simulink model "successPIDCloseLoop21picont"  (R2023b)
settings: Solver=FixedStepAuto  StartTime=0.0  StopTime=inf  RelTol=1e-3  EnableMultiTasking=on
libraries: arduinolib x5, simulink x1, arduinosensorlib x1, slpidlib x1
(part 3 of 3)

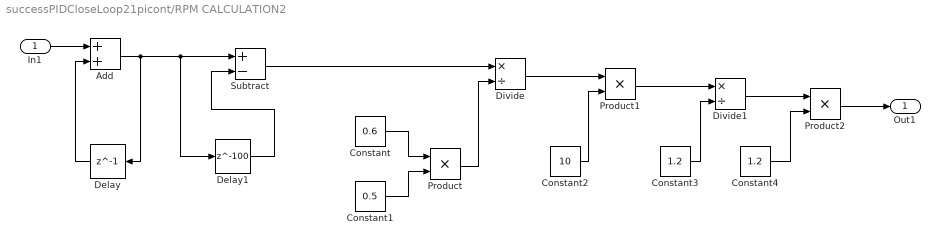
== system successPIDCloseLoop21picont/RPM CALCULATION2 ==
  In1 : Inport
  Add : Sum
  Constant : Constant  Value=0.6  SampleTime=0.001
  Constant1 : Constant  Value=0.5  SampleTime=0.001
  Constant2 : Constant  Value=10  SampleTime=0.001
  Constant3 : Constant  Value=1.2  SampleTime=0.001
  Constant4 : Constant  Value=1.2  SampleTime=0.001
  Delay : Delay  DelayLength=1  InitialCondition=0
  Delay1 : Delay  DelayLength=100  InitialCondition=0
  Divide : Product  Inputs=*/
  Divide1 : Product  Inputs=*/
  Product : Product
  Product1 : Product
  Product2 : Product
  Subtract : Sum  Inputs=+-
  Out1 : Outport
  wires:
  Constant2/1 -> Product1/2
  Product/1 -> Divide/2
  Subtract/1 -> Divide/1
  Product1/1 -> Divide1/1
  Constant4/1 -> Product2/2
  Constant3/1 -> Divide1/2
  Add/1 -> Delay/1, Delay1/1, Subtract/1
  Constant/1 -> Product/1
  Constant1/1 -> Product/2
  Delay/1 -> Add/2
  In1/1 -> Add/1
  Divide/1 -> Product1/1
  Delay1/1 -> Subtract/2
  Divide1/1 -> Product2/1
  Product2/1 -> Out1/1

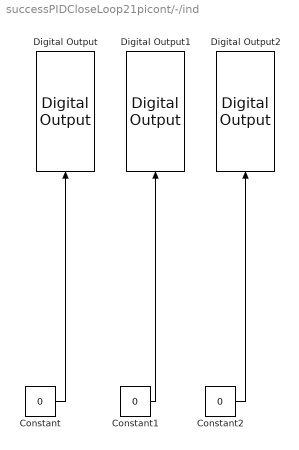
== system successPIDCloseLoop21picont/-/ind ==
  Constant : Constant  Value=0  SampleTime=0.001
  Constant1 : Constant  Value=0  SampleTime=0.001
  Constant2 : Constant  Value=0  SampleTime=0.001
  Digital Output : arduinolib/Digital Output  pinNumber=7  Direction=output  blockPlatform=arduino
  Digital Output1 : arduinolib/Digital Output  pinNumber=8  Direction=output  blockPlatform=arduino
  Digital Output2 : arduinolib/Digital Output  pinNumber=9  Direction=output  blockPlatform=arduino
  wires:
  Constant2/1 -> Digital Output2/1
  Constant/1 -> Digital Output/1
  Constant1/1 -> Digital Output1/1
